simulink model "Piet_Admittance"  (R2016b)
settings: Solver=VariableStepAuto  StartTime=0.0  StopTime=30  RelTol=1e-3
undefined symbols (not defined in the file): b, bh, C, D, dt, J, Jh, JJ, k, K, Ke, kh, M, P
libraries: simulink x2
settings Model: Creator=HumanMechatronics  LastModifiedBy=Com

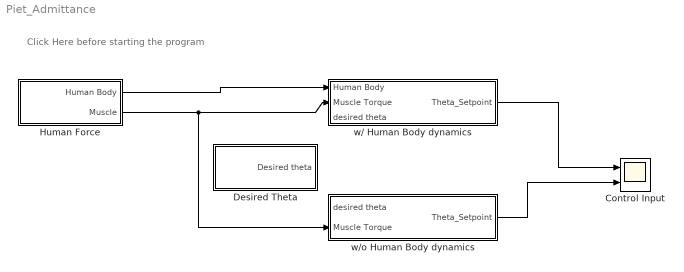
== system Piet_Admittance ==
  note: Click Here before starting the program
  Control Input : Scope  NumInputPorts=2
  Desired Theta : Subsystem
  "Human Force " : Subsystem
  w/ Human Body dynamics : Subsystem
  w/o Human Body dynamics : Subsystem
  wires:
  "Human Force "/2(Muscle) -> w/o Human Body dynamics/2(Muscle Torque), w/ Human Body dynamics/2(Muscle Torque)
  w/ Human Body dynamics/1(Theta_Setpoint) -> Control Input/1
  w/o Human Body dynamics/1(Theta_Setpoint) -> Control Input/2
  "Human Force "/1(Human Body) -> w/ Human Body dynamics/1(Human Body)

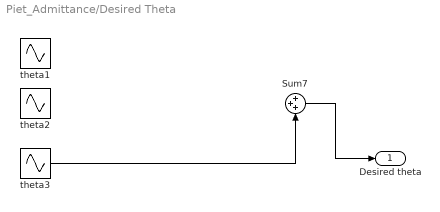
== system Piet_Admittance/Desired Theta ==
  Sum7 : Sum  Inputs=+++
  theta1 : Sin  Amplitude=0.51  Frequency=2*pi*1.21  SampleTime=dt
  theta2 : Sin  Amplitude=1.2  Frequency=2*pi*0.32  SampleTime=dt
  theta3 : Sin  Amplitude=3.5  Frequency=2*pi*0.126
  Desired theta : Outport
  wires:
  Sum7/1 -> Desired theta/1
  theta3/1 -> Sum7/3

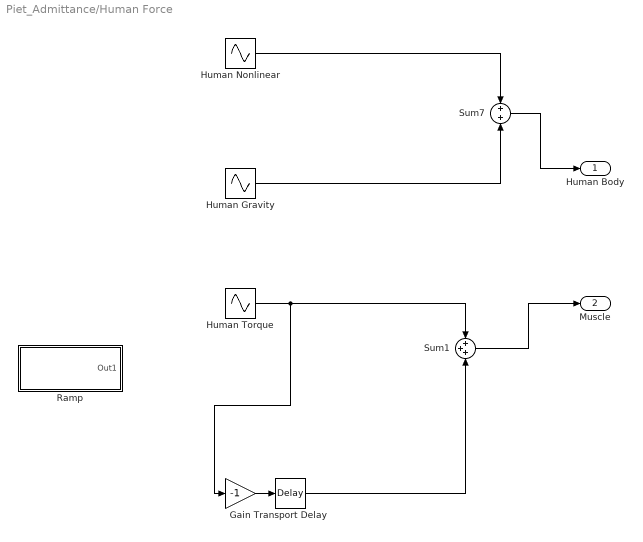
== system Piet_Admittance/Human Force  ==
  Gain : Gain  Gain=-1
  Human Gravity : Sin  Amplitude=7  Frequency=2*pi*0.13
  Human Nonlinear : Sin  Amplitude=1.3  Frequency=2*pi*0.63
  Human Torque : Sin  Amplitude=10  Frequency=2*JJ*pi
  Ramp : Subsystem
  Sum1 : Sum  Inputs=+++
  Sum7 : Sum
  Transport Delay : TransportDelay  DelayTime=3*1/JJ
  Human Body : Outport
  Muscle : Outport  Port=2
  wires:
  Sum7/1 -> Human Body/1
  Sum1/1 -> Muscle/1
  Human Nonlinear/1 -> Sum7/1
  Human Gravity/1 -> Sum7/2
  Human Torque/1 -> Gain/1, Sum1/1
  Gain/1 -> Transport Delay/1
  Transport Delay/1 -> Sum1/3

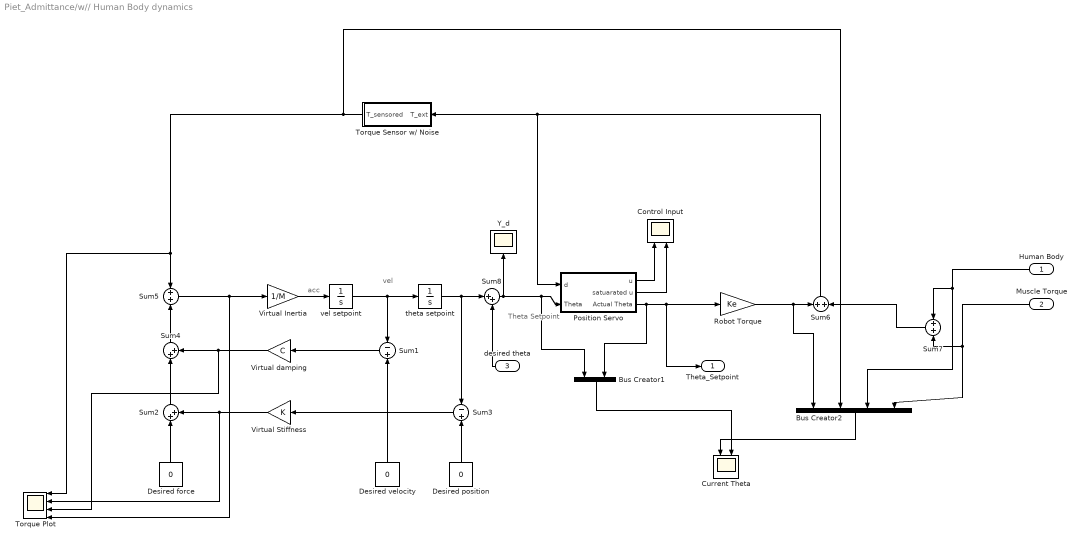
== system Piet_Admittance/w// Human Body dynamics ==
  note: Theta
      | Setpoint
  note: vel
  note: acc
  Human Body : Inport
  Muscle Torque : Inport  Port=2
  desired theta : Inport  Port=3
  Bus Creator1 : BusCreator  Inputs=2
  Bus Creator2 : BusCreator  Inputs=4
  Control Input : Scope  NumInputPorts=2
  Current Theta : Scope  NumInputPorts=2
  Desired force : Constant  Value=0  SampleTime=dt
  Desired position : Constant  Value=0  SampleTime=dt
  Desired velocity : Constant  Value=0  SampleTime=dt
  Position Servo : Subsystem
  Robot Torque : Gain  Gain=Ke
  Sum1 : Sum  Inputs=-|+
  Sum2 : Sum  Inputs=|++
  Sum3 : Sum  Inputs=-|+
  Sum4 : Sum  Inputs=|++
  Sum5 : Sum  Inputs=+|+
  Sum6 : Sum  Inputs=+|+
  Sum7 : Sum
  Sum8 : Sum  Inputs=|++
  Torque Plot : Scope  NumInputPorts=4
  Torque Sensor w/ Noise : Subsystem
  Virtual Inertia : Gain  Gain=1/M
  Virtual Stiffness : Gain  Gain=K
  Virtual damping : Gain  Gain=C
  Y_d : Scope
  theta setpoint : Integrator
  vel setpoint : Integrator
  Theta_Setpoint : Outport
  wires:
  Desired position/1 -> Sum3/2
  Sum3/1 -> Virtual Stiffness/1
  Desired velocity/1 -> Sum1/2
  Sum1/1 -> Virtual damping/1
  Sum2/1 -> Sum4/1
  Virtual Stiffness/1 -> Sum2/2, Torque Plot/2
  Desired force/1 -> Sum2/1
  Virtual damping/1 -> Torque Plot/3, Sum4/2
  Sum4/1 -> Sum5/2
  Virtual Inertia/1 -> vel setpoint/1
  vel setpoint/1 -> theta setpoint/1, Sum1/1
  Position Servo/3(Actual Theta) -> Theta_Setpoint/1, Robot Torque/1, Bus Creator1/2
  Position Servo/1(u) -> Control Input/1
  Position Servo/2(satuarated u) -> Control Input/2
  Bus Creator1/1 -> Current Theta/2
  theta setpoint/1 -> Sum8/1, Sum3/1
  Sum5/1 -> Torque Plot/4, Virtual Inertia/1
  Robot Torque/1 -> Bus Creator2/1, Sum6/1
  Sum6/1 -> Position Servo/1(d), Torque Sensor w/ Noise/1(T_ext)
  Bus Creator2/1 -> Current Theta/1
  Torque Sensor w/ Noise/1(T_sensored) -> Bus Creator2/2, Sum5/1, Torque Plot/1
  Muscle Torque/1 -> Sum7/2, Bus Creator2/4
  Human Body/1 -> Bus Creator2/3, Sum7/1
  Sum7/1 -> Sum6/2
  Sum8/1 -> Y_d/1, Bus Creator1/1, Position Servo/2(Theta)
  desired theta/1 -> Sum8/2

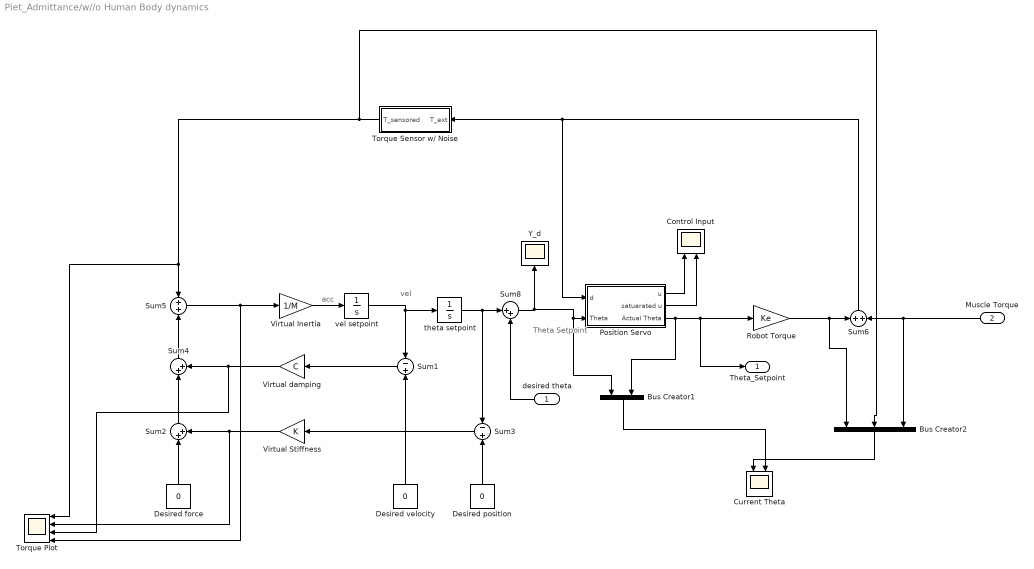
== system Piet_Admittance/w//o Human Body dynamics ==
  note: acc
  note: vel
  note: Theta
      | Setpoint
  desired theta : Inport
  Muscle Torque : Inport  Port=2
  Bus Creator1 : BusCreator  Inputs=2
  Bus Creator2 : BusCreator  Inputs=3
  Control Input : Scope  NumInputPorts=2
  Current Theta : Scope  NumInputPorts=2
  Desired force : Constant  Value=0  SampleTime=dt
  Desired position : Constant  Value=0  SampleTime=dt
  Desired velocity : Constant  Value=0  SampleTime=dt
  Position Servo : Subsystem
  Robot Torque : Gain  Gain=Ke
  Sum1 : Sum  Inputs=-|+
  Sum2 : Sum  Inputs=|++
  Sum3 : Sum  Inputs=-|+
  Sum4 : Sum  Inputs=|++
  Sum5 : Sum  Inputs=+|+
  Sum6 : Sum  Inputs=+|+
  Sum8 : Sum  Inputs=|++
  Torque Plot : Scope  NumInputPorts=4
  Torque Sensor w/ Noise : Subsystem
  Virtual Inertia : Gain  Gain=1/M
  Virtual Stiffness : Gain  Gain=K
  Virtual damping : Gain  Gain=C
  Y_d : Scope
  theta setpoint : Integrator
  vel setpoint : Integrator
  Theta_Setpoint : Outport
  wires:
  Muscle Torque/1 -> Bus Creator2/3, Sum6/2
  Torque Sensor w/ Noise/1(T_sensored) -> Torque Plot/1, Sum5/1, Bus Creator2/2
  Bus Creator2/1 -> Current Theta/1
  Sum6/1 -> Torque Sensor w/ Noise/1(T_ext), Position Servo/1(d)
  Robot Torque/1 -> Sum6/1, Bus Creator2/1
  Sum5/1 -> Virtual Inertia/1, Torque Plot/4
  theta setpoint/1 -> Sum8/1, Sum3/1
  Bus Creator1/1 -> Current Theta/2
  Position Servo/2(satuarated u) -> Control Input/2
  Position Servo/1(u) -> Control Input/1
  Position Servo/3(Actual Theta) -> Bus Creator1/2, Theta_Setpoint/1, Robot Torque/1
  vel setpoint/1 -> Sum1/1, theta setpoint/1
  Virtual Inertia/1 -> vel setpoint/1
  Sum4/1 -> Sum5/2
  Virtual damping/1 -> Sum4/2, Torque Plot/3
  Desired force/1 -> Sum2/1
  Virtual Stiffness/1 -> Torque Plot/2, Sum2/2
  Sum2/1 -> Sum4/1
  Sum1/1 -> Virtual damping/1
  Desired velocity/1 -> Sum1/2
  Sum3/1 -> Virtual Stiffness/1
  Desired position/1 -> Sum3/2
  Sum8/1 -> Bus Creator1/1, Position Servo/2(Theta), Y_d/1
  desired theta/1 -> Sum8/2

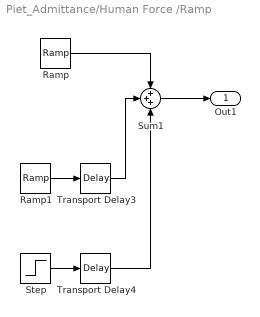
== system Piet_Admittance/Human Force /Ramp ==
  Ramp : simulink/Sources/Ramp  slope=1  start=3  X0=0
  Ramp1 : simulink/Sources/Ramp  slope=-1  start=3  X0=0
  Step : Step  Time=0  After=-10  SampleTime=0
  Sum1 : Sum  Inputs=+++
  Transport Delay3 : TransportDelay  DelayTime=10
  Transport Delay4 : TransportDelay  DelayTime=13
  Out1 : Outport
  wires:
  Ramp/1 -> Sum1/1
  Ramp1/1 -> Transport Delay3/1
  Transport Delay3/1 -> Sum1/2
  Step/1 -> Transport Delay4/1
  Transport Delay4/1 -> Sum1/3
  Sum1/1 -> Out1/1

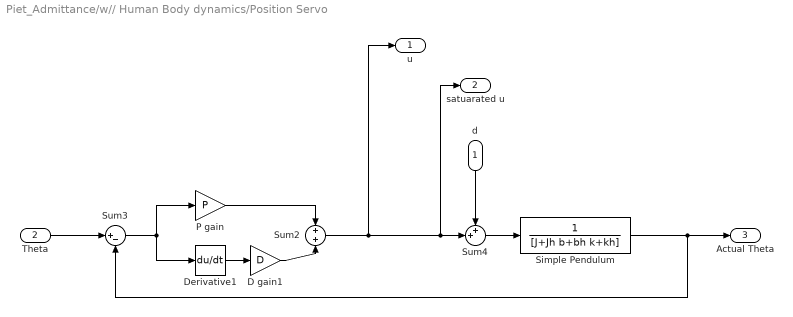
== system Piet_Admittance/w// Human Body dynamics/Position Servo ==
  d : Inport
  Theta : Inport  Port=2
  D gain1 : Gain  Gain=D
  Derivative1 : Derivative
  P gain : Gain  Gain=P
  Simple Pendulum : TransferFcn  Denominator=[J+Jh b+bh k+kh]  ContinuousStateAttributes='Single_Pendulum'
  Sum2 : Sum  Inputs=+|+
  Sum3 : Sum  Inputs=|+-
  Sum4 : Sum  Inputs=++|
  u : Outport
  satuarated u : Outport  Port=2
  Actual Theta : Outport  Port=3
  wires:
  Simple Pendulum/1 -> Sum3/2, Actual Theta/1
  Theta/1 -> Sum3/1
  Sum3/1 -> Derivative1/1, P gain/1
  d/1 -> Sum4/1
  Sum4/1 -> Simple Pendulum/1
  Sum2/1 -> satuarated u/1, Sum4/2, u/1
  Derivative1/1 -> D gain1/1
  P gain/1 -> Sum2/1
  D gain1/1 -> Sum2/2

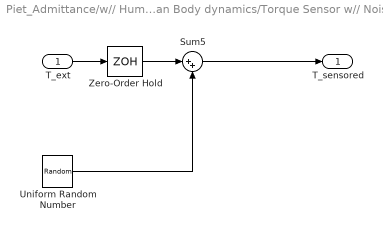
== system Piet_Admittance/w// Human Body dynamics/Torque Sensor w// Noise ==
  T_ext : Inport
  Sum5 : Sum  Inputs=|++
  Uniform Random Number : UniformRandomNumber  Minimum=-0.5  Maximum=0.5  SampleTime=0.005
  Zero-Order Hold : ZeroOrderHold  SampleTime=dt
  T_sensored : Outport
  wires:
  Zero-Order Hold/1 -> Sum5/1
  T_ext/1 -> Zero-Order Hold/1
  Sum5/1 -> T_sensored/1
  Uniform Random Number/1 -> Sum5/2

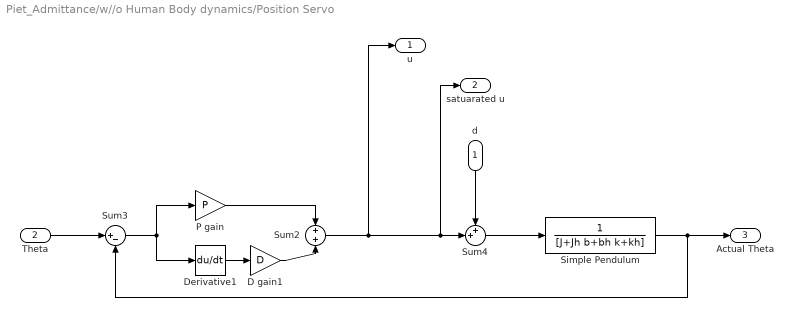
== system Piet_Admittance/w//o Human Body dynamics/Position Servo ==
  d : Inport
  Theta : Inport  Port=2
  D gain1 : Gain  Gain=D
  Derivative1 : Derivative
  P gain : Gain  Gain=P
  Simple Pendulum : TransferFcn  Denominator=[J+Jh b+bh k+kh]  ContinuousStateAttributes='Single_Pendulum'
  Sum2 : Sum  Inputs=+|+
  Sum3 : Sum  Inputs=|+-
  Sum4 : Sum  Inputs=++|
  u : Outport
  satuarated u : Outport  Port=2
  Actual Theta : Outport  Port=3
  wires:
  D gain1/1 -> Sum2/2
  P gain/1 -> Sum2/1
  Derivative1/1 -> D gain1/1
  Sum2/1 -> u/1, Sum4/2, satuarated u/1
  Sum4/1 -> Simple Pendulum/1
  d/1 -> Sum4/1
  Sum3/1 -> P gain/1, Derivative1/1
  Theta/1 -> Sum3/1
  Simple Pendulum/1 -> Actual Theta/1, Sum3/2

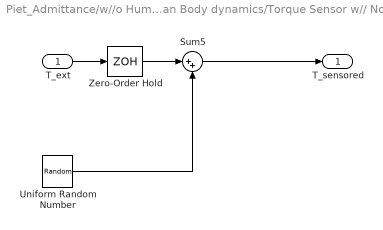
== system Piet_Admittance/w//o Human Body dynamics/Torque Sensor w// Noise ==
  T_ext : Inport
  Sum5 : Sum  Inputs=|++
  Uniform Random Number : UniformRandomNumber  Minimum=-0.5  Maximum=0.5  SampleTime=0.005
  Zero-Order Hold : ZeroOrderHold  SampleTime=dt
  T_sensored : Outport
  wires:
  Sum5/1 -> T_sensored/1
  T_ext/1 -> Zero-Order Hold/1
  Zero-Order Hold/1 -> Sum5/1
  Uniform Random Number/1 -> Sum5/2
